simulink model "iv_v_DetectObject"  (R2023b)
settings: Solver=FixedStepDiscrete  StartTime=0.0  StopTime=60  FixedStep=0.01  RelTol=1e-3
undefined symbols (not defined in the file or in its folder): DiscIntNeverNeededParam
libraries: arduinolib x16, simulink x14, mobileRoboticsTrainingLib x1, arduinosensorlib x1
settings Model: SimulationMode=accelerator  NumberOfSteps=10  SnapshotBufferSize=20  ExtModeTrigDuration=2  Creator=Boitumelo  LastModifiedBy=cameronclark
settings OptimizationCC: EnhancedBackFolding=on  PassReuseOutputArgsAs=Individual arguments  ZeroExternalMemoryAtStartup=off  ZeroInternalMemoryAtStartup=off  MaxStackSize=64  OptimizeBlockOrder=speed  DifferentSizesBufferReuse=on  OptimizationCustomize=off  EfficientTunableParamExpr=on
settings DebuggingCC: ParameterTunabilityLossMsg=error  UnconnectedInputMsg=warning  UnconnectedOutputMsg=warning  UnconnectedLineMsg=warning
settings HardwareCC: ProdBitPerPointer=32  ProdBitPerSizeT=32  ProdBitPerPtrDiffT=32  ProdLargestAtomicInteger=Long  ProdLargestAtomicFloat=Double  ProdWordSize=32  ProdHWDeviceType=ARM Compatible->ARM Cortex  UseEmbeddedCoderFeatures=off  UseSimulinkCoderFeatures=off
settings ModelReferenceCC: EnableRefExpFcnMdlSchedulingChecks=on
settings SFSimCC: MATLABDynamicMemAlloc=off
settings RTWCC: Description=Embedded Coder  SystemTargetFile=ert.tlc  HardwareBoard=Arduino Nano 33 IoT  TemplateMakefile=ert_default_tmf  Toolchain=Arduino ARM  BuildConfiguration=Faster Runs  DLArmComputeVersion=19.05
settings CodeAppCC: ForceParamTrailComments=on  IgnoreCustomStorageClasses=off  OperatorAnnotations=on  SimulinkDataObjDesc=on  SFDataObjDesc=on  InsertBlockDesc=on
settings ERTTargetCC: SupportContinuousTime=on  SupportNonInlinedSFcns=on  SupportVariableSizeSignals=on  ExtModeTransport=3  ExtModeStaticAlloc=on  ExtModeAutomaticAllocSize=off  ExtModeStaticAllocSize=8192  ExtModeMexFile=ext_xcp  ExtModeIntrfLevel=Level2 - Open

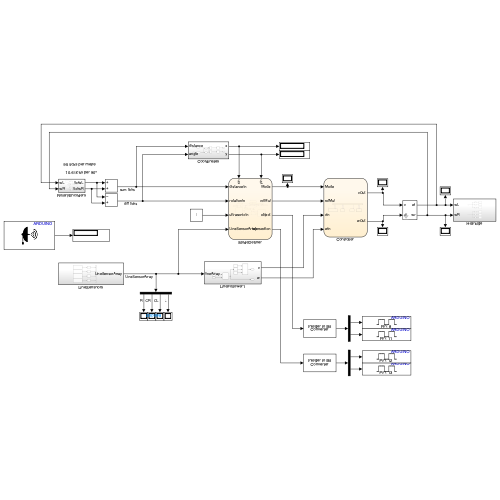
[thumbnail: Simulink's stored preview of the top-level diagram]
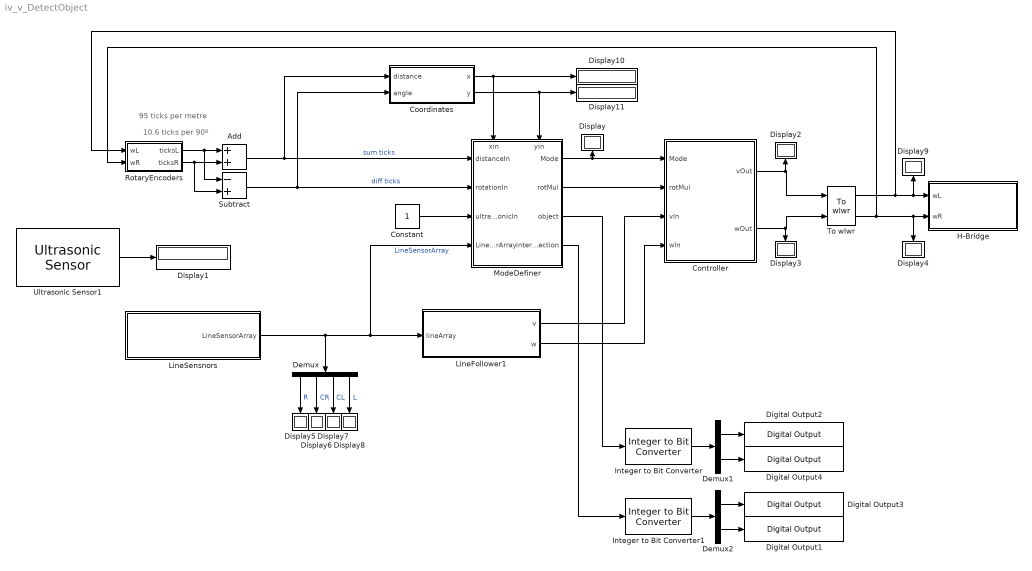
== system iv_v_DetectObject ==
  note: 10.6 ticks per 90º
  note: 95 ticks per metre
  Add : Sum
  Constant : Constant
  Controller : Stateflow chart  TreatAsAtomicUnit=on
      settings: PortSchema="{\"entries\":[{\"content\":{\"sides\":[{\"content\":{\"connectorIds\":[\"In2\",\"In1\",\"In3\",\"In4\"]},\"type\":\"ConnectorPlacement.EquallySpacedRectSide\",\"uuid\":\"0e13ea10-b264-4fbc-ab83-bc41241a6c36\"},{\"content\":{\"connectorIds\":[\"Out1\",\"Out2\"],\"side\":\"RIGHT\"},\"type\":\"ConnectorPlacement.EquallySpacedRectSide\",\"uuid\":\"9cddfb1b-e196-4e58-b952-6299e40de404\"},{\"content\":{\"side\":\"TOP\"},\"type\":\"ConnectorPlacement.EquallySpacedRectSide\",\"uuid\":\"e3e699c2-e489-41cc-aace-e70cb50311af\"}]},\"type\":\"ConnectorPlacement.EquallySpacedConnector\",\"uuid\":\"1d087cfb-49f0-41b6-92be-dfee541679f3\"}],\"packageUris\":[\"http://schema.mathworks.com/mf0/Connector/R2020b\"],\"version\":\"1.0\"}"
  Coordinates : Subsystem
  Demux : Demux
  Demux1 : Demux  Outputs=2
  Demux2 : Demux  Outputs=2
  Digital Output1 : arduinolib/Digital Output  pinNumber=13  Direction=output  blockPlatform=arduino
  Digital Output2 : arduinolib/Digital Output  pinNumber=8  Direction=output  blockPlatform=arduino
  Digital Output3 : arduinolib/Digital Output  pinNumber=12  Direction=output  blockPlatform=arduino
  Digital Output4 : arduinolib/Digital Output  pinNumber=11  Direction=output  blockPlatform=arduino
  Display{,1..11} (12 alike) : Display
  H-Bridge : Subsystem
  Integer to Bit Converter : simulink/Logic and Bit Operations/Integer to Bit Converter  nbits=2  signedInputValues=Unsigned  bitOrder=MSB first  outDtype=Inherit via internal rule
  Integer to Bit Converter1 : simulink/Logic and Bit Operations/Integer to Bit Converter  nbits=2  signedInputValues=Unsigned  bitOrder=MSB first  outDtype=Inherit via internal rule
  LineFollower1 : Subsystem
  LineSensnors : Subsystem
  ModeDefiner : Stateflow chart  TreatAsAtomicUnit=on
      settings: PortSchema="{\"entries\":[{\"content\":{\"sides\":[{\"content\":{\"connectorIds\":[\"In4\",\"In5\",\"In3\",\"In6\"]},\"type\":\"ConnectorPlacement.EquallySpacedRectSide\",\"uuid\":\"2e12269d-ccd1-4e68-8415-629d2e368e6d\"},{\"content\":{\"connectorIds\":[\"Out1\",\"Out2\",\"Out3\",\"Out4\"],\"side\":\"RIGHT\"},\"type\":\"ConnectorPlacement.EquallySpacedRectSide\",\"uuid\":\"1564c0f6-61d7-475f-9f3f-a1f2c1915817\"},{\"content\":{\"connectorIds\":[\"In1\",\"In2\"],\"side\":\"TOP\"},\"type\":\"ConnectorPlacement.EquallySpacedRectSide\",\"uuid\":\"729d5d21-cc85-429f-97c7-0630790832c8\"}]},\"type\":\"ConnectorPlacement.EquallySpacedConnector\",\"uuid\":\"65fad4a7-698e-4a16-b156-07c77b4027bb\"}],\"packageUris\":[\"http://schema.mathworks.com/mf0/Connector/R2020b\"],\"version\":\"1.0\"}"
  RotaryEncoders : Subsystem
  Subtract : Sum  Inputs=-+
  To wlwr : mobileRoboticsTrainingLib/To wlwr  axleLength=0.14  wheelR=0.033
      link override change parameters: Gain=[1 -axleLength/2;1 axleLength/2]
  Ultrasonic Sensor1 : arduinosensorlib/Ultrasonic Sensor  NumSignalPins=2  TrigPin=0  EchoPin=1  SignalPin=3  SampleTime_=1  blockPlatform=ARDUINO
  wires:
  LineSensnors/1(LineSensorArray) -> Demux/1, LineFollower1/1(lineArray), ModeDefiner/6(LineSensorArray)  "LineSensorArray"
  LineFollower1/2(w) -> Controller/4(wIn)
  Controller/1(vOut) -> To wlwr/1, Display2/1
  Controller/2(wOut) -> Display3/1, To wlwr/2
  LineFollower1/1(v) -> Controller/3(vIn)
  Demux/1 -> Display5/1  "R"
  Demux/2 -> Display6/1  "CR"
  Demux/4 -> Display8/1  "L"
  Demux/3 -> Display7/1  "CL"
  ModeDefiner/1(Mode) -> Display/1, Controller/2(Mode)
  ModeDefiner/2(rotMul) -> Controller/1(rotMul)
  Coordinates/1(x) -> Display10/1, ModeDefiner/1(xin)
  Coordinates/2(y) -> Display11/1, ModeDefiner/2(yin)
  To wlwr/1 -> RotaryEncoders/1(wL), Display9/1, H-Bridge/1(wL)
  To wlwr/2 -> RotaryEncoders/2(wR), Display4/1, H-Bridge/2(wR)
  RotaryEncoders/1(ticksL) -> Subtract/1, Add/1
  RotaryEncoders/2(ticksR) -> Subtract/2, Add/2
  Add/1 -> Coordinates/1(distance), ModeDefiner/4(distanceIn)  "sum ticks"
  Subtract/1 -> Coordinates/2(angle), ModeDefiner/5(rotationIn)  "diff ticks"
  Ultrasonic Sensor1/1 -> Display1/1
  Constant/1 -> ModeDefiner/3(ultrasonicIn)
  Demux2/1 -> Digital Output3/1
  Integer to Bit Converter/1 -> Demux1/1
  Demux1/1 -> Digital Output2/1
  Demux1/2 -> Digital Output4/1
  ModeDefiner/3(object) -> Integer to Bit Converter/1
  Demux2/2 -> Digital Output1/1
  Integer to Bit Converter1/1 -> Demux2/1
  ModeDefiner/4(intersection) -> Integer to Bit Converter1/1

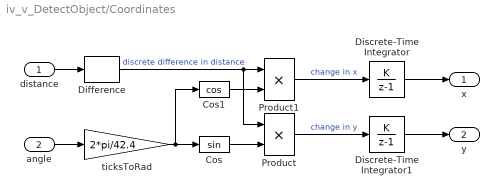
== system iv_v_DetectObject/Coordinates ==
  distance : Inport
  angle : Inport  Port=2
  Cos : Trigonometry
  Cos1 : Trigonometry  Operator=cos
  Difference : simulink/Discrete/Difference  ICPrevInput=0.0  InputProcessing=Columns as channels (frame based)  OutMin=[]  OutMax=[]  OutDataType=fixdt(1, 16)  OutScaling=2^-10  DoSatur=off
  Discrete-Time Integrator : DiscreteIntegrator  IntegratorMethod=Accumulation: Forward Euler  gainval=1  SampleTime=-1  ICPrevOutput=DiscIntNeverNeededParam  ICPrevScaledInput=DiscIntNeverNeededParam
  Discrete-Time Integrator1 : DiscreteIntegrator  IntegratorMethod=Accumulation: Forward Euler  gainval=1  SampleTime=-1  ICPrevOutput=DiscIntNeverNeededParam  ICPrevScaledInput=DiscIntNeverNeededParam
  Product : Product
  Product1 : Product
  ticksToRad : Gain  Gain=2*pi/42.4
  x : Outport
  y : Outport  Port=2
  wires:
  distance/1 -> Difference/1
  Difference/1 -> Product1/1, Product/1  "discrete difference in distance"
  Product/1 -> Discrete-Time Integrator1/1  "change in y"
  Product1/1 -> Discrete-Time Integrator/1  "change in x"
  angle/1 -> ticksToRad/1
  ticksToRad/1 -> Cos/1, Cos1/1
  Cos/1 -> Product/2
  Cos1/1 -> Product1/2
  Discrete-Time Integrator/1 -> x/1
  Discrete-Time Integrator1/1 -> y/1

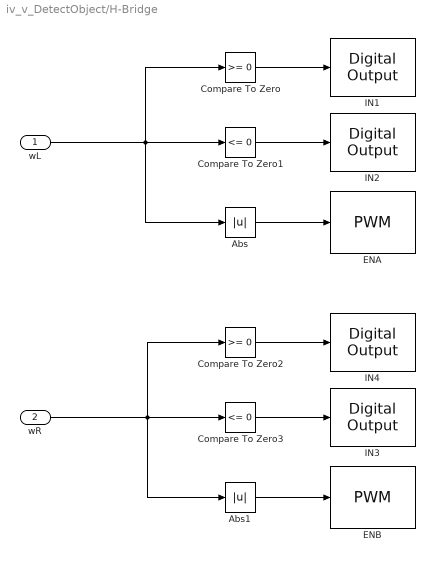
== system iv_v_DetectObject/H-Bridge ==
  wL : Inport
  wR : Inport  Port=2
  Abs : Abs  SaturateOnIntegerOverflow=off
  Abs1 : Abs  SaturateOnIntegerOverflow=off
  Compare To Zero : simulink/Logic and Bit Operations/Compare To Zero  relop=>=  OutDataTypeStr=boolean
  Compare To Zero1 : simulink/Logic and Bit Operations/Compare To Zero  relop=<=  OutDataTypeStr=boolean
  Compare To Zero2 : simulink/Logic and Bit Operations/Compare To Zero  relop=>=  OutDataTypeStr=boolean
  Compare To Zero3 : simulink/Logic and Bit Operations/Compare To Zero  relop=<=  OutDataTypeStr=boolean
  ENA : arduinolib/PWM  pinNumber=4  frequencyType=Default  desiredFrequency=490.2  achievableFrequency=490.2
  ENB : arduinolib/PWM  pinNumber=5  frequencyType=Default  desiredFrequency=490.2  achievableFrequency=490.2
  IN1 : arduinolib/Digital Output  pinNumber=2  Direction=output  blockPlatform=arduino
  IN2 : arduinolib/Digital Output  pinNumber=3  Direction=output  blockPlatform=arduino
  IN3 : arduinolib/Digital Output  pinNumber=7  Direction=output  blockPlatform=arduino
  IN4 : arduinolib/Digital Output  pinNumber=6  Direction=output  blockPlatform=arduino
  wires:
  Compare To Zero1/1 -> IN2/1
  Compare To Zero/1 -> IN1/1
  Abs1/1 -> ENB/1
  Compare To Zero3/1 -> IN3/1
  Compare To Zero2/1 -> IN4/1
  wL/1 -> Compare To Zero/1, Compare To Zero1/1, Abs/1
  Abs/1 -> ENA/1
  wR/1 -> Compare To Zero2/1, Compare To Zero3/1, Abs1/1

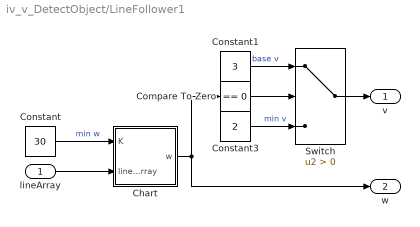
== system iv_v_DetectObject/LineFollower1 ==
  lineArray : Inport
  Chart : Stateflow chart  TreatAsAtomicUnit=on
  Compare To Zero : simulink/Logic and Bit Operations/Compare To Zero  relop===  OutDataTypeStr=boolean
  Constant : Constant  Value=30
  Constant1 : Constant  Value=3
  Constant3 : Constant  Value=2
  Switch : Switch  Criteria=u2 > Threshold  SaturateOnIntegerOverflow=off  InputSameDT=off
  v : Outport
  w : Outport  Port=2
  wires:
  Constant1/1 -> Switch/1  "base v"
  Chart/1(w) -> Compare To Zero/1, w/1
  Constant3/1 -> Switch/3  "min v"
  Switch/1 -> v/1
  lineArray/1 -> Chart/2(lineArray)
  Compare To Zero/1 -> Switch/2
  Constant/1 -> Chart/1(K)  "min w"

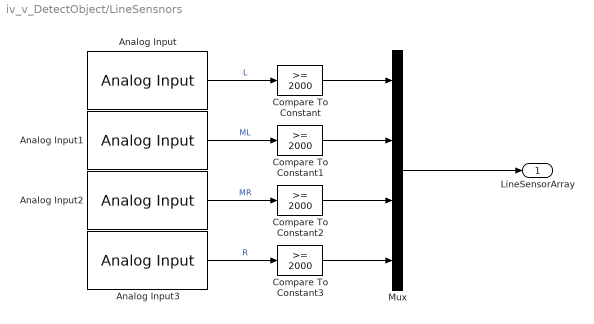
== system iv_v_DetectObject/LineSensnors ==
  Analog Input : arduinolib/Analog Input  pinNumber=7  ReadResultsOnly=off  ConversionTriggerSource=Software  ExternalTriggerType=uint32( 0 )  OutputDataType=uint16  EnableConversionCompleteNotify=off  EnableOuputStatus=off  SampleTime=-1  blockPlatform=arduino
  Analog Input1 : arduinolib/Analog Input  pinNumber=6  ReadResultsOnly=off  ConversionTriggerSource=Software  ExternalTriggerType=uint32( 0 )  OutputDataType=uint16  EnableConversionCompleteNotify=off  EnableOuputStatus=off  SampleTime=-1  blockPlatform=arduino
  Analog Input2 : arduinolib/Analog Input  pinNumber=3  ReadResultsOnly=off  ConversionTriggerSource=Software  ExternalTriggerType=uint32( 0 )  OutputDataType=uint16  EnableConversionCompleteNotify=off  EnableOuputStatus=off  SampleTime=-1  blockPlatform=arduino
  Analog Input3 : arduinolib/Analog Input  pinNumber=2  ReadResultsOnly=off  ConversionTriggerSource=Software  ExternalTriggerType=uint32( 0 )  OutputDataType=uint16  EnableConversionCompleteNotify=off  EnableOuputStatus=off  SampleTime=-1  blockPlatform=arduino
  Compare To Constant{,1..3} (4 alike) : simulink/Logic and Bit Operations/Compare To Constant  relop=>=  const=2000  OutDataTypeStr=boolean
  Mux : Mux
  LineSensorArray : Outport
  wires:
  Mux/1 -> LineSensorArray/1
  Analog Input/1 -> Compare To Constant/1  "L"
  Analog Input1/1 -> Compare To Constant1/1  "ML"
  Analog Input2/1 -> Compare To Constant2/1  "MR"
  Analog Input3/1 -> Compare To Constant3/1  "R"
  Compare To Constant/1 -> Mux/1
  Compare To Constant1/1 -> Mux/2
  Compare To Constant2/1 -> Mux/3
  Compare To Constant3/1 -> Mux/4

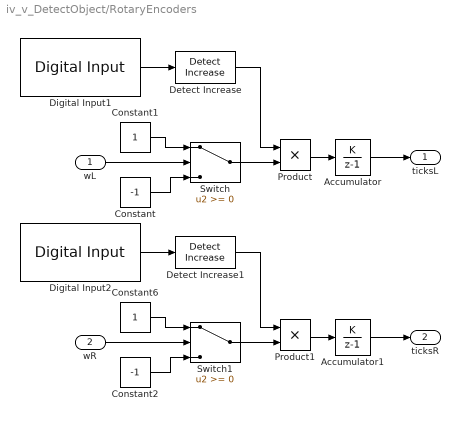
== system iv_v_DetectObject/RotaryEncoders ==
  wL : Inport
  wR : Inport  Port=2
  Accumulator : DiscreteIntegrator  IntegratorMethod=Accumulation: Forward Euler  SampleTime=-1  ICPrevOutput=DiscIntNeverNeededParam  ICPrevScaledInput=DiscIntNeverNeededParam
  Accumulator1 : DiscreteIntegrator  IntegratorMethod=Accumulation: Forward Euler  SampleTime=-1  ICPrevOutput=DiscIntNeverNeededParam  ICPrevScaledInput=DiscIntNeverNeededParam
  Constant : Constant  Value=-1
  Constant1 : Constant
  Constant2 : Constant  Value=-1
  Constant6 : Constant
  Detect Increase : simulink/Logic and Bit Operations/Detect Increase  vinit=0.0  OutDataTypeStr=boolean
  Detect Increase1 : simulink/Logic and Bit Operations/Detect Increase  vinit=0.0  OutDataTypeStr=boolean
  Digital Input1 : arduinolib/Digital Input  pinNumber=9  mode=Default  Direction=input  SampleTime=0.1  blockPlatform=arduino
  Digital Input2 : arduinolib/Digital Input  pinNumber=10  mode=Default  Direction=input  SampleTime=0.1  blockPlatform=arduino
  Product : Product
  Product1 : Product
  Switch : Switch  SaturateOnIntegerOverflow=off  InputSameDT=off
  Switch1 : Switch  SaturateOnIntegerOverflow=off  InputSameDT=off
  ticksL : Outport
  ticksR : Outport  Port=2
  wires:
  wL/1 -> Switch/2
  Constant1/1 -> Switch/1
  Constant/1 -> Switch/3
  Digital Input1/1 -> Detect Increase/1
  Switch/1 -> Product/2
  Accumulator/1 -> ticksL/1
  wR/1 -> Switch1/2
  Constant6/1 -> Switch1/1
  Constant2/1 -> Switch1/3
  Accumulator1/1 -> ticksR/1
  Switch1/1 -> Product1/2
  Product/1 -> Accumulator/1
  Detect Increase/1 -> Product/1
  Detect Increase1/1 -> Product1/1
  Digital Input2/1 -> Detect Increase1/1
  Product1/1 -> Accumulator1/1

== stateflow chart iv_v_DetectObject/ModeDefiner ==
  state Start
    entry:
    Mode = 0; %Drive
    intersections = -1 * ones(5,3,4) %[x y;angle1-4;visited1-4]
    intersection = 1; %the last index of the intersections array
    currentIntersection = 1; %the intersection the robot is at
    objects = -1 * ones(5, 4); %[x y distance rotation]
    object = 1; %last index of the objects array
    stopZoneFound = 0;
    defaultPath=2 %the path to take if there are no unexplored paths on current intersection
  state RotateBackToLine
    entry:
    Mode = 4;
    rotMul = rotMul * -1;
    exit:
    Mode = 0;
  state Explore
    %Go forth and find the next thing
  state DriveAwayFromInterrupt
    entry:
    Mode = 0;
    distanceTarget = distanceIn + 4;
  state RotateToLine
    entry:
    if (LineSensorArray(1) == 0)
    rotMul = 1;
    else
    rotMul = -1;
    end
    Mode = 4;
  state TurnAround
    entry:
    Mode = 4;
    rotationTarget = rotationIn + 21;
    rotMul = 1;
  state RecordObject
    entry:
    objects(object,:) = [xin yin ultrasonicIn rotationIn];
    object = object + 1;
  state DriveBackToLine
    entry:
    Mode = 0;
    distanceTarget = distanceIn + 6
  state CentreOnIntersection
    entry:
    %rot mul determines the direction of the rotation
    if (LineSensorArray(1) == 0)
    rotMul = 1;
    else
    rotMul = -1;
    end
    distanceTarget = distanceIn + 6;
  state SenseNewIntersection
    entry:
    Mode = 4; % rotate
    if all(LineSensorArray(2:3)==0) %is there an intersection infront
    rotationTarget = 0; %assume that robot is at an intersection
    else
    %the robot might be just off the line, so if it has to rotate less than 45° to find a line
    %return to the path
    rotationTarget = rotationIn + 5*rotMul;
    end
    rotationHalf = rotationIn + 21*rotMul; %half rotatation target
    rotationFull = rotationIn + 42*rotMul; %full rotation target
    lineSensorRising = 2.5 - 0.5*rotMul; %the rising edge line sensor
    lineSensorFalling = 2.5 + 0.5*rotMul; %the falling edge line sensor
    %when detecting a line, one sensor will have a rising edge, and one will have a falling edge,
    %take the average of those two angles will give the angle of the intersection
    risingEdge = LineSensorArray(lineSensorRising);
    fallingEdge = LineSensorArray(lineSensorFalling);
    fallingEdgeDetected = 0;
    rotationFalling = 0;
    path = 1;
    if (~LineSensorArray(2) | ~LineSensorArray(3))
    %robot is facing a path to start with
    intersections(intersection,2,path) = rotationIn;
    intersections(intersection,3,path) = 0;
    path = path + 1;
    end
    during:
    if rotationTarget
    if (rotMul*(rotationTarget-rotationIn) >= 0) & all(LineSensorArray(2:3)==0)
    %robot rotated less than 45° and is back on path, thus, no intersection
    Mode = 1;
    end
    end
    if fallingEdge & ~LineSensorArray(lineSensorFalling)
    rotationFalling = rotationIn; %initial side of a path detected
    fallingEdgeDetected = 1;
    end
    if ~risingEdge & LineSensorArray(lineSensorRising)
    if fallingEdgeDetected
    %other side of the intersection
    intersections(intersection,2,path) = (rotationIn + rotationFalling)/2;
    fallingEdgeDetected = 0;
    if rotationHalf & (abs(intersections(intersection,2,path) - rotationHalf) <= 3)
    %180° rotated thus, it is the path we came from, mark as return path.
    intersections(intersection,3,path) = 2 + stopZoneFound;
    rotationHalf = 0;
    else
    %else mark as unexplored
    intersections(intersection,3,path) = 0;
    end
    path = path + 1;
    end
    end
    %updating edges
    risingEdge = LineSensorArray(lineSensorRising);
    fallingEdge = LineSensorArray(lineSensorFalling);
  state Stop
    entry:
    Mode = 3;
  state PickPath
    entry:
    Mode = 4;
    if stopZoneFound %stop zone found so mark path that returns to stop zone
    if ~any(intersections(currentIntersection,3,:)==3)
    for path = 1:4
    if abs(abs(mod(intersections(currentIntersection,2,path)-rotationIn,42))-21) <= 3
    intersections(currentIntersection,3,path) = 3;
    break;
    end
    end
    end
    end
    if any(intersections(currentIntersection,3,:)==0)
    %there is an unexplored path so take it
    for path = 4:-1:1
    if ~intersections(currentIntersection,3,path)
    intersections(currentIntersection,3,path) = 1;
    rotationTarget = intersections(currentIntersection,2,path)
    if rotationTarget-rotationIn > 0
    rotMul = 1;
    else
    rotMul = -1;
    end
    break;
    end
    end
    else
    %go back down return path OR stop zone path if no unexplored paths left
    for path = 1:4
    if intersections(currentIntersection,3,path)==defaultPath
    rotationTarget = intersections(currentIntersection,2,path)
    if rotationTarget-rotationIn > 0
    rotMul = 1;
    else
    rotMul = -1;
    end
    break
    end
    end
    end
  state CheckForOldIntersection
    entry:
    %checks if the x y of the robot match any x y of any recorded intersections
    oldIntersection = 0;
    for currentIntersection = 1:5
    if ~all(intersections(currentIntersection,3,:)==-1)
    if abs(intersections(currentIntersection,1,1)-xin) <= 9
    if abs(intersections(currentIntersection,1,2)-yin) <= 9
    oldIntersection = 1;
    break;
    end
    end
    end
    end
  state AddIntersection
    entry:
    %next intersection in array
    intersections(intersection,1,1) = xin;
    intersections(intersection,1, 2) = yin;
    currentIntersection = intersection;
    intersection = intersection + 1;
  (default) -> Start
  Start -> Explore
  RotateBackToLine -> Explore : [all(LineSensorArray(2:3)==0)]
  DriveBackToLine -> RotateBackToLine : [distanceIn>=distanceTarget]
  Explore -> (junction 118) [order 1] : [(LineSensorArray(1) == 0) | (LineSensorArray(4) == 0)]%interrupt triggered
  DriveAwayFromInterrupt -> Explore : [distanceIn >= distanceTarget]
  Explore -> TurnAround [order 2] : [all(LineSensorArray==1)]
      | %at a dead end
  TurnAround -> DriveAwayFromInterrupt : [rotationIn>rotationTarget]
  RecordObject -> TurnAround
  (junction 118) -> RotateToLine [order 3] : [all(LineSensorArray(2:3)==1)]
      | %Robot is off the line
  (junction 118) -> RecordObject [order 1] : [ultrasonicIn & (ultrasonicIn <= 0.5)]
      | %at measurement line
  (junction 118) -> CentreOnIntersection [order 2] : [(LineSensorArray(1) == 0) & (LineSensorArray(4) == 0)]
      | %At a T intersection
  (junction 118) -> CentreOnIntersection [order 4] : %default: assume at intersection
  PickPath -> DriveAwayFromInterrupt : [rotMul*(rotationTarget-rotationIn) <= 0]
      | %rotated to target path
  RotateToLine -> DriveBackToLine : [all(LineSensorArray(2:3)==0)]
  (junction 99) -> TurnAround [order 1] : [any(any(intersections(:,3,:) == 0))]{stopZoneFound =1;}
      | %There are unexplore paths, return to them
  SenseNewIntersection -> DriveBackToLine [order 1] : [Mode==1]
      | %continue back to path
  CentreOnIntersection -> (junction 93) : [distanceIn >= distanceTarget]
  (junction 93) -> (junction 99) [order 1] : [all(LineSensorArray==0)]
      | %At a stop zone not an intersection
  (junction 93) -> CheckForOldIntersection [order 2] : %default: at intersection
  (junction 99) -> Stop [order 2] : %All paths explored
  CheckForOldIntersection -> SenseNewIntersection [order 1] : [~oldIntersection]
  (junction 113) -> PickPath [order 1] : [any(any(intersections(:,3,:)==0))]{defaultPath=2;}
      | %there are still unexplored intersections
      | %thus, go down the return intersections
  CheckForOldIntersection -> (junction 113) [order 2] : [oldIntersection]
      | %this intersection has been found
  (junction 113) -> PickPath [order 2] : {defaultPath=3;}
      | %there are no unexplored intersections
      | %thus, return to stop zone
  AddIntersection -> PickPath
  SenseNewIntersection -> AddIntersection [order 2] : [(abs(rotationIn - rotationFull) <= 2)]{defaultPath==2}
      | %fully rotated so intersection recorded
  data: xin input; yin input; ultrasonicIn input; Mode output =0; rotMul output; distanceIn input; distanceTarget local; rotationIn input; LineSensorArray input; fallingEdge local; rotationHalf local; rotationFull local; path local; rotationTarget local; risingEdge local; lineSensorFalling local; lineSensorRising local; rotationFalling local; fallingEdgeDetected local; intersections local; oldIntersection local; currentIntersection local; stopZoneFound local; defaultPath local; objects local; object output; intersection output

== stateflow chart iv_v_DetectObject/Controller ==
  state StartBlock
  state Rotate
    during:
    wOut = 30*rotMul;
    vOut = 0;
  state Drive %using LineFollow algorithm
    during:
    wOut = wIn;
    vOut = vIn;
  state DriveForward
    entry:
    wOut = 0;
    vOut = 2;
  state Stop
    en:
    vOut=0;
    wOut=0;
  Drive %using LineFollow algorithm -> StartBlock : [Mode~=0]
  StartBlock -> Drive %using LineFollow algorithm [order 1] : [Mode==0]
  DriveForward -> StartBlock : [Mode~=1]
  StartBlock -> DriveForward [order 4] : [Mode==1]
  StartBlock -> Stop [order 3] : [Mode==3]
  Rotate -> StartBlock : [Mode~=4]
  StartBlock -> Rotate [order 2] : [Mode==4]
  (default) -> Drive %using LineFollow algorithm
  data: rotMul input; Mode input; vIn input; wIn input; vOut output; wOut output

== stateflow chart iv_v_DetectObject/LineFollower1/Chart ==
  state ComputeW
    %code for the line array
    during:
    w = K*(lineArray(3)-lineArray(2));
  (default) -> ComputeW
  data: w output; K input; lineArray input
